simulink model "SMIB_sim"  (Simulink 8.3)
settings: Solver=ode45  StartTime=0.0  StopTime=Time  FixedStep=1e-4  MaxStep=1e-2  RelTol=1e-4
values from neighbouring files (symbols this model uses):
  D = 20    [RUNTHIS.m]    (also in optimization.m; pso.m; test.m; test_with_pss.m)
  dTm = 0.20    (= 0.2)    [RUNTHIS.m]    (also in optimization.m; pso.m; test.m; test_with_pss.m)
  dVref = 0.0    (= 0)    [RUNTHIS.m]    (also in optimization.m; pso.m; test.m; test_with_pss.m)
  H = 3.25    [RUNTHIS.m]    (also in optimization.m; pso.m; test.m; test_with_pss.m)
  K1 = (-1/DELTA)*(Iq0*Vinf*(Xpd-Xq)*((Xq+Xe)*sin(delta0)-Re*cos(delta0))+         Vinf*((Xpd-Xq)*Id0-Epq0)*((Xpd+Xe)*cos(delta0)+Re*sin(delta0)))    [RUNTHIS.m]    (also in optimization.m = (-1/DELTA)*(Iq0*Vinf*(Xpd-Xq)*((Xq+Xe)*sin(delta0)-Re*cos(de; pso.m = (-1/DELTA)*(Iq0*Vinf*(Xpd-Xq)*((Xq+Xe)*sin(delta0)-Re*cos(de; test.m = (-1/DELTA)*(Iq0*Vinf*(Xpd-Xq)*((Xq+Xe)*sin(delta0)-Re*cos(de; test_with_pss.m = (-1/DELTA)*(Iq0*Vinf*(Xpd-Xq)*((Xq+Xe)*sin(delta0)-Re*cos(de)
  K2 = (1/DELTA)*(Iq0*DELTA-Iq0*(Xpd-Xq)*(Xq+Xe)-Re*(Xpd-Xq)*Id0+Re*Epq0)    [RUNTHIS.m]    (also in optimization.m; pso.m; test.m; test_with_pss.m)
  K3 = 1/(1+((Xd-Xpd)*(Xq+Xe)/DELTA))    (= 0.272413793103)    [RUNTHIS.m]    (also in optimization.m = 0.296666666667; pso.m = 0.296666666667; test.m = 0.296666666667; test_with_pss.m = 0.296666666667)
  K4 = (Vinf*(Xd-Xpd)/DELTA)*((Xq+Xe)*sin(delta0)-Re*cos(delta0))    [RUNTHIS.m]    (also in optimization.m; pso.m; test.m; test_with_pss.m)
  K5 = (1/DELTA)*((Vd0/abs(Vt0))*Xq*(Re*Vinf*sin(delta0)+Vinf*cos(delta0)*         (Xpd+Xe))+(Vq0/abs(Vt0))*(Xpd*(Re*Vinf*cos(delta0)-Vinf*(Xq+Xe)*         sin(delta0))))    [RUNTHIS.m]    (also in optimization.m = (1/DELTA)*((Vd0/abs(Vt0))*Xq*(Re*Vinf*sin(delta0)+Vinf*cos(d; pso.m = (1/DELTA)*((Vd0/abs(Vt0))*Xq*(Re*Vinf*sin(delta0)+Vinf*cos(d; test.m = (1/DELTA)*((Vd0/abs(Vt0))*Xq*(Re*Vinf*sin(delta0)+Vinf*cos(d; test_with_pss.m = (1/DELTA)*((Vd0/abs(Vt0))*Xq*(Re*Vinf*sin(delta0)+Vinf*cos(d)
  K6 = (1/DELTA)*((Vd0/abs(Vt0))*Xq*Re-(Vq0/abs(Vt0))*Xpd*(Xq+Xe))+         (Vq0/abs(Vt0))    [RUNTHIS.m]    (also in optimization.m = (1/DELTA)*((Vd0/abs(Vt0))*Xq*Re-(Vq0/abs(Vt0))*Xpd*(Xq+Xe))+; pso.m = (1/DELTA)*((Vd0/abs(Vt0))*Xq*Re-(Vq0/abs(Vt0))*Xpd*(Xq+Xe))+; test.m = (1/DELTA)*((Vd0/abs(Vt0))*Xq*Re-(Vq0/abs(Vt0))*Xpd*(Xq+Xe))+; test_with_pss.m = (1/DELTA)*((Vd0/abs(Vt0))*Xq*Re-(Vq0/abs(Vt0))*Xpd*(Xq+Xe))+)
  KA = 400    [RUNTHIS.m]    (also in optimization.m; pso.m; test.m; test_with_pss.m)
  Kpss = Ub1    [RUNTHIS.m]    (also in optimization.m = bestOrganism(1); pso.m = GlobalBest.Position(3); test.m = bestOrganism(1); test_with_pss.m = bestOrganism(1))
  PSS = 1    [optimization.m]    (also in pso.m; test.m = 0; test_with_pss.m = 0)
  T = 3    [optimization.m]    (also in pso.m; test.m; test_with_pss.m)
  T1 = Ub2    [RUNTHIS.m]    (also in optimization.m = bestOrganism(2); pso.m = GlobalBest.Position(1); test.m = bestOrganism(2); test_with_pss.m = bestOrganism(2))
  T2 = Ub3    [RUNTHIS.m]    (also in optimization.m = bestOrganism(3); pso.m = GlobalBest.Position(2); test.m = bestOrganism(3); test_with_pss.m = bestOrganism(3))
  TA = 0.2    [RUNTHIS.m]    (also in optimization.m; pso.m; test.m; test_with_pss.m)
  Tpdo = 9.6    [RUNTHIS.m]    (also in optimization.m; pso.m; test.m; test_with_pss.m)
  tsim = 1.0005    [RUNTHIS.m]    (also in optimization.m; pso.m; test.m; test_with_pss.m)
  ws = 377    [RUNTHIS.m]    (also in optimization.m; pso.m; test.m; test_with_pss.m)
settings Model: Creator=sevim  LastModifiedBy=Munmun
settings DataIOCC: SignalLoggingSaveFormat=Dataset
settings GRTTargetCC: CombineOutputUpdateFcns=on  GRTInterface=off

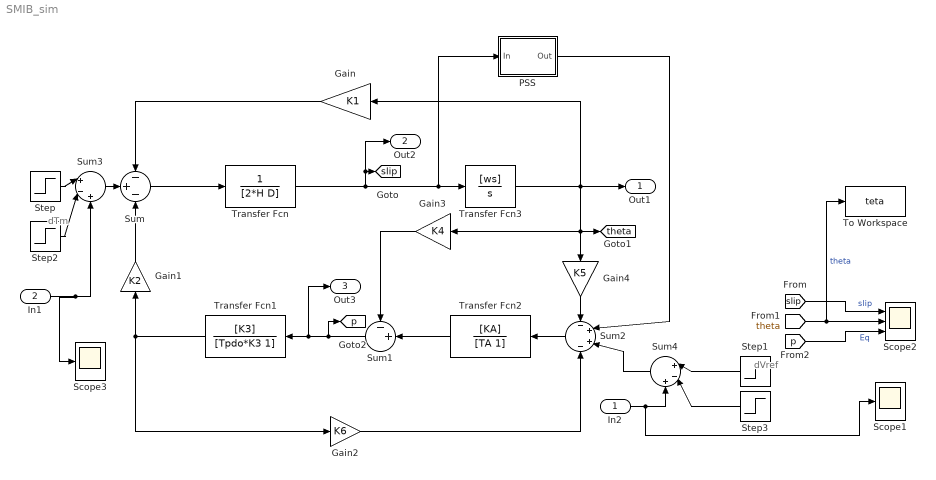
== system SMIB_sim ==
  note: dTm
  note: dVref
  In2 : Inport
  In1 : Inport  Port=2
  Gain : Gain  Gain=K1
  Gain1 : Gain  Gain=K2
  Gain2 : Gain  Gain=K6
  Gain3 : Gain  Gain=K4
  Gain4 : Gain  Gain=K5
  PSS : Subsystem
  Scope1 : Scope
      settings: YMin=-0.000838014  YMax=-0.000758204  MaxDataPoints=50000000
  Scope2 : Scope  NumInputPorts=3
      settings: YMin=-0.000838014~-0.428567~-5  YMax=-0.000758204~-0.387751~5  SaveName=ScopeData2  MaxDataPoints=50000000
  Scope3 : Scope
      settings: YMin=-0.000838014  YMax=-0.000758204  MaxDataPoints=50000000
  Step : Step  After=dTm  SampleTime=0
  Step1 : Step  After=dVref  SampleTime=0
  Step2 : Step  Time=tsim  After=dTm  SampleTime=0
  Step3 : Step  Time=tsim  After=dVref  SampleTime=0
  Sum : Sum  Inputs=-+-
  Sum1 : Sum  Inputs=-+|
  Sum2 : Sum  Inputs=-++-
  Sum3 : Sum  Inputs=|+-+
  Sum4 : Sum  Inputs=|+-+
  To Workspace : ToWorkspace  VariableName=teta  SampleTime=-1
  Transfer Fcn : TransferFcn  Denominator=[2*H D]
  Transfer Fcn1 : TransferFcn  Numerator=[K3]  Denominator=[Tpdo*K3 1]
  Transfer Fcn2 : TransferFcn  Numerator=[KA]  Denominator=[TA 1]
  Transfer Fcn3 : TransferFcn  Numerator=[ws]  Denominator=[1 0]
  Out1 : Outport
  Out2 : Outport  Port=2
  Out3 : Outport  Port=3
  tag scope: p=global, slip=global, theta=global
  wires:
  Sum/1 -> Transfer Fcn/1
  Gain/1 -> Sum/1
  Gain1/1 -> Sum/3
  Transfer Fcn1/1 -> Gain2/1, Gain1/1
  Sum1/1 -> [p], Out3/1, Transfer Fcn1/1
  Transfer Fcn2/1 -> Sum1/2
  Gain3/1 -> Sum1/1
  Sum2/1 -> Transfer Fcn2/1
  Transfer Fcn/1 -> Out2/1, [slip], PSS/1(In), Transfer Fcn3/1
  Gain4/1 -> Sum2/1
  Transfer Fcn3/1 -> [theta], Gain4/1, Gain3/1, Out1/1, Gain/1
  [slip] -> Scope2/1  "slip"
  [theta] -> To Workspace/1, Scope2/2  "theta"
  Gain2/1 -> Sum2/4
  Sum4/1 -> Sum2/3
  [p] -> Scope2/3  "Eq"
  Step/1 -> Sum3/1
  Step2/1 -> Sum3/2
  Step1/1 -> Sum4/1
  Step3/1 -> Sum4/2
  Sum3/1 -> Sum/2
  In2/1 -> Scope1/1, Sum4/3
  In1/1 -> Scope3/1, Sum3/3
  PSS/1(Out) -> Sum2/2

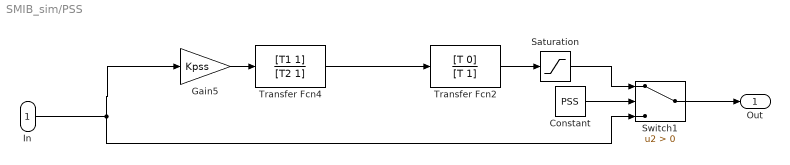
== system SMIB_sim/PSS ==
  In : Inport
  Constant : Constant  Value=PSS
  Gain5 : Gain  Gain=Kpss
  Saturation : Saturate  UpperLimit=0.2  LowerLimit=-0.2
  Switch1 : Switch  Criteria=u2 > Threshold
  Transfer Fcn2 : TransferFcn  Numerator=[T 0]  Denominator=[T 1]
  Transfer Fcn4 : TransferFcn  Numerator=[T1 1]  Denominator=[T2 1]
  Out : Outport
  wires:
  Gain5/1 -> Transfer Fcn4/1
  Transfer Fcn4/1 -> Transfer Fcn2/1
  In/1 -> Gain5/1, Switch1/3
  Switch1/1 -> Out/1
  Saturation/1 -> Switch1/1
  Constant/1 -> Switch1/2
  Transfer Fcn2/1 -> Saturation/1
